simulink model "HW2_2_disc_5"  (R2021a)
settings: Solver=VariableStepAuto  StartTime=0.0  StopTime=2  RelTol=1e-3
settings Model: Creator=jhart  LastModifiedBy=jhart

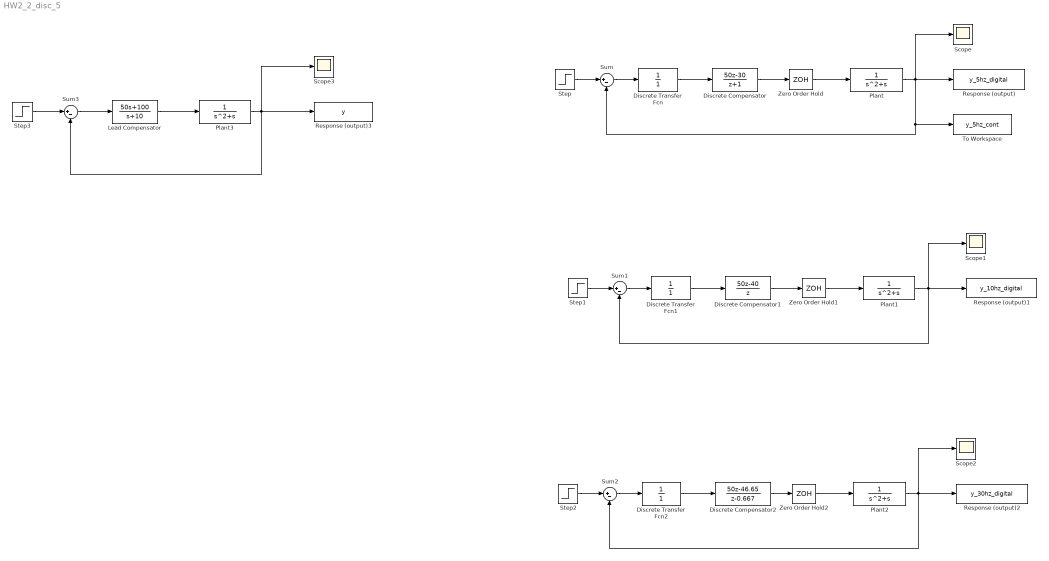
== system HW2_2_disc_5 ==
  Discrete Transfer Fcn : DiscreteTransferFcn  Denominator=[1]  SampleTime=0.2
  Discrete Transfer Fcn1 : DiscreteTransferFcn  Denominator=[1]  SampleTime=0.1
  Discrete Transfer Fcn2 : DiscreteTransferFcn  Denominator=[1]  SampleTime=0.033
  Discrete Compensator : DiscreteTransferFcn  Numerator=[50 -30]  Denominator=[1 1]  SampleTime=0.2
  Discrete Compensator1 : DiscreteTransferFcn  Numerator=[50 -40]  Denominator=[1 0]  SampleTime=0.1
  Discrete Compensator2 : DiscreteTransferFcn  Numerator=[50 -46.65]  Denominator=[1 -0.667]  SampleTime=0.033
  Lead Compensator : TransferFcn  Numerator=[50 100]  Denominator=[1 10]
  Plant{,1..3} (4 alike) : TransferFcn  Denominator=[1 1 0]
  Response (output) : ToWorkspace  VariableName=y_5hz_digital  SaveFormat=Timeseries  SampleTime=0.2
  Response (output)1 : ToWorkspace  VariableName=y_10hz_digital  SaveFormat=Timeseries  SampleTime=0.1
  Response (output)2 : ToWorkspace  VariableName=y_30hz_digital  SaveFormat=Timeseries  SampleTime=0.033
  Response (output)3 : ToWorkspace  VariableName=y  SaveFormat=Timeseries  SampleTime=-1
  Scope{,1..3} (4 alike) : Scope
  Step{,1..3} (4 alike) : Step  Time=0  SampleTime=0
  Sum{,1..3} (4 alike) : Sum  Inputs=|+-
  To Workspace : ToWorkspace  VariableName=y_5hz_cont  SaveFormat=Timeseries  SampleTime=-1
  Zero Order Hold : ZeroOrderHold  SampleTime=0.2
  Zero Order Hold1 : ZeroOrderHold  SampleTime=0.1
  Zero Order Hold2 : ZeroOrderHold  SampleTime=0.033
  wires:
  Plant/1 -> Sum/2, To Workspace/1, Response (output)/1, Scope/1
  Discrete Compensator/1 -> Zero Order Hold/1
  Step/1 -> Sum/1
  Zero Order Hold/1 -> Plant/1
  Sum/1 -> Discrete Transfer Fcn/1
  Discrete Transfer Fcn/1 -> Discrete Compensator/1
  Discrete Transfer Fcn1/1 -> Discrete Compensator1/1
  Zero Order Hold1/1 -> Plant1/1
  Plant1/1 -> Scope1/1, Sum1/2, Response (output)1/1
  Step1/1 -> Sum1/1
  Sum1/1 -> Discrete Transfer Fcn1/1
  Discrete Compensator1/1 -> Zero Order Hold1/1
  Sum2/1 -> Discrete Transfer Fcn2/1
  Step2/1 -> Sum2/1
  Discrete Compensator2/1 -> Zero Order Hold2/1
  Zero Order Hold2/1 -> Plant2/1
  Discrete Transfer Fcn2/1 -> Discrete Compensator2/1
  Plant2/1 -> Scope2/1, Sum2/2, Response (output)2/1
  Plant3/1 -> Scope3/1, Sum3/2, Response (output)3/1
  Lead Compensator/1 -> Plant3/1
  Sum3/1 -> Lead Compensator/1
  Step3/1 -> Sum3/1
